simulink model "IM200HP_Test_Model"  (Simulink 8.1)
settings: Solver=ode4  StartTime=0.0  StopTime=100  FixedStep=Ts  RelTol=1e-3
PostLoadFcn:
  | Ts=1000e-6;
InitFcn:
  | Ts=1000e-6;
libraries: powerlib x4, ModifiedInductionMachine_lib x1, breaker_lib x1
settings Model: Creator=ed12083  LastModifiedBy=RE25624
settings DataIOCC: SignalLoggingSaveFormat=Dataset
settings OptimizationCC: ExpressionDepthLimit=128
settings DebuggingCC: FcnCallInpInsideContextMsg=EnableAllAsError
settings GRTTargetCC: CombineOutputUpdateFcns=on  GRTInterface=off

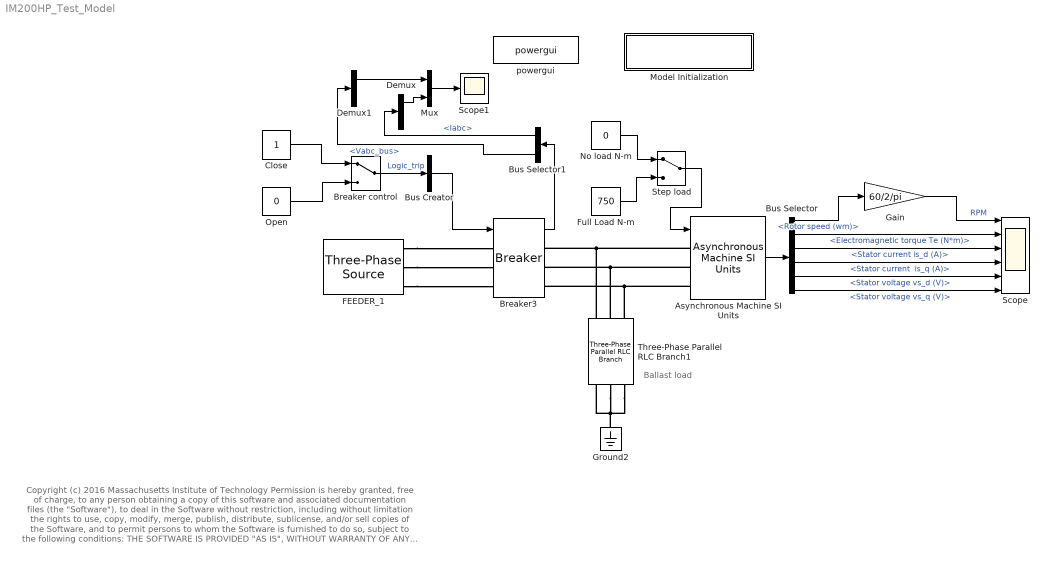
== system IM200HP_Test_Model ==
  note: Ballast load
  note: Copyright (c) 2016 Massachusetts Institute of Technology
      | Permission is hereby granted, free of charge, to any person obtaining a copy of this software and associated documentation files (the "Software"), to deal
      | in the Software without restriction, including without limitation the rights to use, copy, modify, merge, publish, distribute, sublicense, and/or sell copies of the
      | Software, and to permit persons to whom the Software is furnished to do so, subject to the following conditions:
      |
      | THE SOFTWARE IS PROVIDED "AS IS", WITHOUT WARRANTY OF ANY KIND, EXPRESS OR IMPLIED, INCLUDING BUT NOT LIMITED TO THE
      | WARRANTIES OF MERCHANTABILITY, FITNESS FOR A PARTICULAR PURPOSE AND NONINFRINGEMENT. IN NO EVENT SHALL THE AUTHORS
      | OR COPYRIGHT HOLDERS BE LIABLE FOR ANY CLAIM, DAMAGES OR OTHER LIABILITY, WHETHER IN AN ACTION OF CONTRACT, TORT OR
      | OTHERWISE, ARISING FROM, OUT OF OR IN CONNECTION WITH THE SOFTWARE OR THE USE OR OTHER DEALINGS IN THE SOFTWARE.
  Asynchronous Machine SI Units : ModifiedInductionMachine_lib/Asynchronous Machine SI Units  PresetModel=No  MechanicalLoad=Torque Tm  ShowDetailedParameters=on  RotorType=Squirrel-cage  ReferenceFrame=Stationary  NominalParameters=[ 136700/.92/.93, 480, 60 ]  Stator=[ 0.029 0.226/377/1.5]  Rotor=[ 0.022*3 0.226/377/1.5]  Cage1=[ 0.022 0.226/377]  Cage2=[ 0.022 0.226/377]  Lm=13.04/377  Mechanical="[ 63.87 0  2 ]"  PolePairs=2  InitialConditions=[1 0 0 0 0 0 0 0]  Units=SI  LoadFlowParameters=1492000  SimulateSaturation=off  Saturation=[14.03593122, 27.81365428, 53.79336849, 72.68890987, 97.98006896, 148.6815601, 215.7428561, 302.9841135, 420.4778367 ; 230, 322, 414, 460, 506, 552, 598, 644, 690]  TsPowergui=0  TsBlock=-1  IterativeModel=Trapezoidal non iterative  Pmec=0
      settings: AttributesFormatString=\n
  Breaker control : ManualSwitch
  Breaker3 : breaker_lib/Breaker  Ts=Ts
  Bus Creator : BusCreator  Inputs=1
  Bus Selector : BusSelector  OutputSignals="Mechanical.Rotor speed (wm),Mechanical.Electromagnetic torque Te (N*m),Stator measurements.Stator current is_d (A),Stator measurements.Stator current  is_q (A),Stator measurements.Stator voltage vs_d (V),Stator measurements.Stator voltage vs_q (V)"
  Bus Selector1 : BusSelector  OutputSignals=Iabc,Vabc_bus
  Close : Constant
  Demux : Demux  Outputs=3
  Demux1 : Demux  Outputs=3
  FEEDER_1 : powerlib/Electrical Sources/Three-Phase Source  Voltage=480  PhaseAngle=0  Frequency=60  InternalConnection=Yg  SpecifyImpedance=on  Resistance=0.8929  Inductance=16.58e-3  ShortCircuitLevel=375e6  BaseVoltage=480  XRratio=7.9  BusType=swing  Pref=0  Qref=0  Qmin=-inf  Qmax=inf
  Full Load N-m : Constant  Value=750
  Gain : Gain  Gain=60/2/pi
  Ground2 : powerlib/Elements/Ground  LConnTagsString=a
  Model Initialization : Subsystem  AncestorBlock=artemis/Tools /Misc/Model Initialization  mask(Model Functions){InitFcnX=Ts=1000e-6;, prel=off, posl=on, inif=on, strf=off}
      mask prompts: InitFcnX "Initialisation"; prel "Preload Function"; posl "PostLoad Function"; inif "InitFcn"; strf "StartFcn"
      mask init:
      | currentBlock = gcb;
      | root = bdroot(currentBlock);
      | 
      | if ~strcmp(get_param(root,'BlockDiagramType'),'library')
      |     if prel==1
      |         set_param(root, 'PreLoadFcn', InitFcnX);
      |     else
      |         set_param(root, 'PreLoadFcn', '');
      |     end
      |     if inif==1
      |         set_param(root, 'InitFcn', InitFcnX);
      |     else
      |         set_param(root, 'InitFcn', '');
      |     end
      |     if strf==1
      |         set_param(root, 'StartFcn', InitFcnX);
      |     else
      |         set_param(root, 'StartFcn', '');
      |     end
      |     if posl==1
      |         set_param(root, 'PostLoadFcn', InitFcnX);
      |     else
      |         set_param(root, 'PostLoadFcn', '');
      |     end
      | end
      | 
      | pos = get_param(currentBlock, 'Position');
      | width = pos(3) - pos(1); height = pos(4) - pos(2);
      | txt = [ upper(root) '\n' '- InitFcn. . . . . '  get_param(root, 'InitFcn') ];
      settings: CopyFcn=set_param(gcb,'LinkStatus','inactive')
      mask Display: text(5, height*0.5, txt, 'horizontalAlignment', 'left', 'verticalAlignment', 'middle') ;
  Mux : Mux  Inputs=2
  No load N-m : Constant  Value=0
  Open : Constant  Value=0
  Scope : Scope  NumInputPorts=6
      settings: YMin=-250~-2000~-1500~-1250~-400~-400  YMax=2000~4000~1250~1500~400~400
  Scope1 : Scope
  Step load : ManualSwitch
  Three-Phase Parallel RLC Branch1 : powerlib/Elements/Three-Phase Parallel RLC Branch  LConnTagsString=A|B|C  RConnTagsString=A|B|C  BranchType=RLC  Resistance=1e6  Inductance=inf  Capacitance=0  Measurements=None
  powergui : powerlib/powergui  Priority=2  SimulationMode=Discrete  SolverType=Tustin  SampleTime=Ts  frequency=60  SPID=off  DisableSnubberDevices=off  DisableRonSwitches=off  DisableVfSwitches=off  SwTol=0  Interpol=off  DisplayEquations=off  frequencyindice=0  Pbase=100e6  ErrMax=1e-4  Iterations=50  UnitsV=kV  UnitsW=MW  FunctionMessages=off  echomessages=off  HookPort=off  EnableUseOfTLC=off  x0status=blocks  RestoreLinks=warning  ResistiveCurrentMeasurement=off  Frange=logspace(0,3,50)  Ylog=off  Xlog=off  ShowGrid=off  save=off  variable=ZData  structure=0  ZoomFFT=on  StartTime=0.0  cycles=2  DisplayStyle=off  fundamental=60  FreqAxis=off  MaxFrequency=1000  frequencyindicesteady=1  RmsSteady=1  display=off  Ts=0  methode=off
  wires:
  Breaker control/1 -> Bus Creator/1  "Logic_trip"
  Bus Creator/1 -> Breaker3/1
  Close/1 -> Breaker control/1
  Open/1 -> Breaker control/2
  Step load/1 -> Asynchronous Machine SI Units/1
  Asynchronous Machine SI Units/1 -> Bus Selector/1
  Bus Selector/1 -> Gain/1  "<Rotor speed (wm)>"
  Bus Selector/2 -> Scope/2  "<Electromagnetic torque Te (N*m)>"
  Bus Selector/3 -> Scope/3  "<Stator current is_d (A)>"
  Bus Selector/4 -> Scope/4  "<Stator current  is_q (A)>"
  Bus Selector/5 -> Scope/5  "<Stator voltage vs_d (V)>"
  Bus Selector/6 -> Scope/6  "<Stator voltage vs_q (V)>"
  Gain/1 -> Scope/1  "RPM"
  Full Load N-m/1 -> Step load/2
  No load N-m/1 -> Step load/1
  Breaker3/1 -> Bus Selector1/1
  Bus Selector1/1 -> Demux/1  "<Iabc>"
  Bus Selector1/2 -> Demux1/1  "<Vabc_bus>"
  Mux/1 -> Scope1/1
  Demux/1 -> Mux/2
  Demux1/1 -> Mux/1
  connections:
  Three-Phase Parallel RLC Branch1/RConn1 -- Asynchronous Machine SI Units/LConn1 -- Breaker3/RConn1
  Three-Phase Parallel RLC Branch1/RConn2 -- Asynchronous Machine SI Units/LConn2 -- Breaker3/RConn2
  Three-Phase Parallel RLC Branch1/RConn3 -- Asynchronous Machine SI Units/LConn3 -- Breaker3/RConn3
  FEEDER_1/RConn1 -- Breaker3/LConn1
  FEEDER_1/RConn2 -- Breaker3/LConn2
  FEEDER_1/RConn3 -- Breaker3/LConn3
  Ground2/LConn1 -- Three-Phase Parallel RLC Branch1/LConn3 -- Three-Phase Parallel RLC Branch1/LConn2 -- Three-Phase Parallel RLC Branch1/LConn1

== system IM200HP_Test_Model/Model Initialization ==
